simulink model "Weight_Extract_IQRD_RLS_model_top_8x8"  (R2020b)
settings: Solver=VariableStepAuto  StartTime=0.0  StopTime=0.00001  RelTol=1e-3
settings Model: Creator=jgentile  LastModifiedBy=jgentile

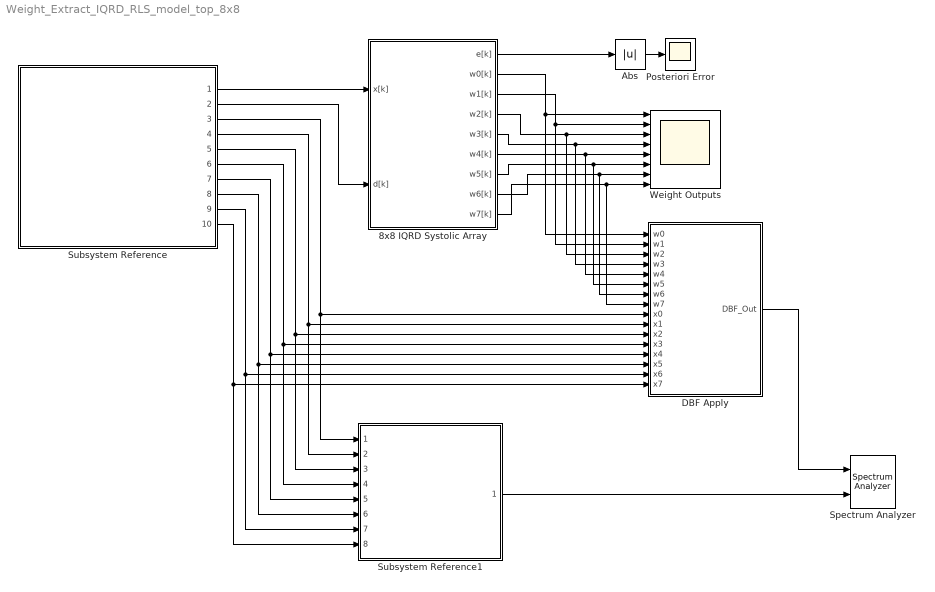
== system Weight_Extract_IQRD_RLS_model_top_8x8 ==
  8x8 IQRD Systolic Array : Subsystem
  Abs : Abs
  DBF Apply : Subsystem
  Posteriori Error : Scope
  Spectrum Analyzer : SpectrumAnalyzer  NumInputPorts=2
  Subsystem Reference : Subsystem  ReferencedSubsystem=s8x8_ULA_additive_Noise_Interference
  Subsystem Reference1 : Subsystem  ReferencedSubsystem=Weighted_Sum_Avg_No_ABF_8x8
  Weight Outputs : Scope  NumInputPorts=8
  wires:
  Subsystem Reference/1 -> 8x8 IQRD Systolic Array/1(x[k])
  Subsystem Reference/2 -> 8x8 IQRD Systolic Array/2(d[k])
  8x8 IQRD Systolic Array/2(w0[k]) -> DBF Apply/1(w0), Weight Outputs/1
  8x8 IQRD Systolic Array/3(w1[k]) -> DBF Apply/2(w1), Weight Outputs/2
  8x8 IQRD Systolic Array/4(w2[k]) -> DBF Apply/3(w2), Weight Outputs/3
  Subsystem Reference1/1 -> Spectrum Analyzer/2
  DBF Apply/1(DBF_Out) -> Spectrum Analyzer/1
  Abs/1 -> Posteriori Error/1
  Subsystem Reference/3 -> DBF Apply/9(x0), Subsystem Reference1/1
  Subsystem Reference/4 -> DBF Apply/10(x1), Subsystem Reference1/2
  Subsystem Reference/5 -> DBF Apply/11(x2), Subsystem Reference1/3
  Subsystem Reference/6 -> DBF Apply/12(x3), Subsystem Reference1/4
  Subsystem Reference/7 -> DBF Apply/13(x4), Subsystem Reference1/5
  Subsystem Reference/8 -> DBF Apply/14(x5), Subsystem Reference1/6
  Subsystem Reference/9 -> DBF Apply/15(x6), Subsystem Reference1/7
  Subsystem Reference/10 -> DBF Apply/16(x7), Subsystem Reference1/8
  8x8 IQRD Systolic Array/1(e[k]) -> Abs/1
  8x8 IQRD Systolic Array/5(w3[k]) -> DBF Apply/4(w3), Weight Outputs/4
  8x8 IQRD Systolic Array/6(w4[k]) -> DBF Apply/5(w4), Weight Outputs/5
  8x8 IQRD Systolic Array/7(w5[k]) -> DBF Apply/6(w5), Weight Outputs/6
  8x8 IQRD Systolic Array/8(w6[k]) -> DBF Apply/7(w6), Weight Outputs/7
  8x8 IQRD Systolic Array/9(w7[k]) -> DBF Apply/8(w7), Weight Outputs/8

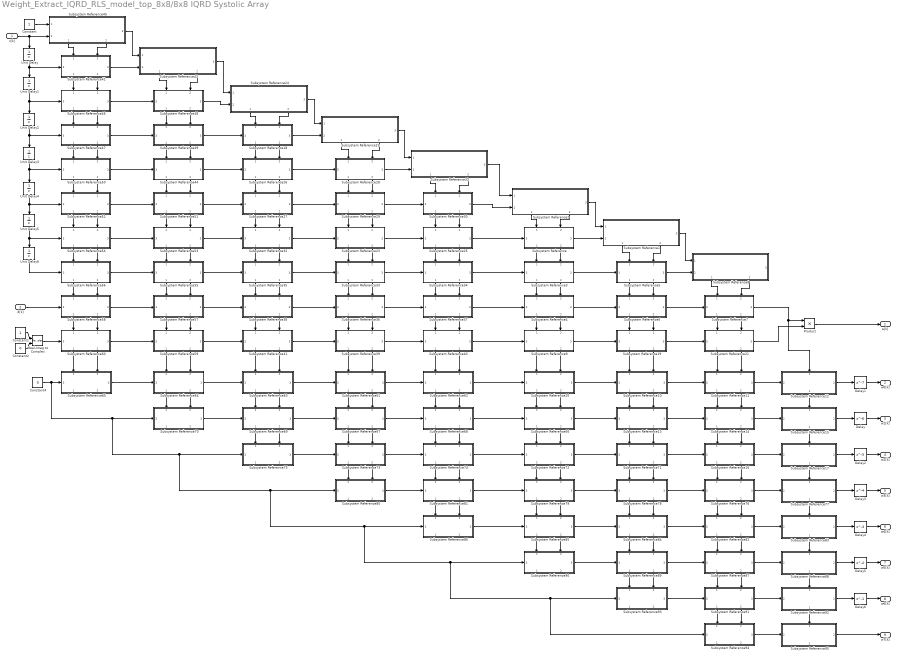
== system Weight_Extract_IQRD_RLS_model_top_8x8/8x8 IQRD Systolic Array ==
  x[k] : Inport
  d[k] : Inport  Port=2
  Constant : Constant
  Constant1 : Constant
  Constant2 : Constant  Value=0
  Constant4 : Constant  Value=0
  Delay : Delay  DelayLength=6
  Delay1 : Delay  DelayLength=7
  Delay2 : Delay  DelayLength=5
  Delay3 : Delay  DelayLength=4
  Delay4 : Delay  DelayLength=3
  Delay5 : Delay
  Delay6 : Delay  DelayLength=1
  Product : Product
  Real-Imag to Complex : RealImagToComplex
  Subsystem Reference{,3..7,9,18..19,21,23,25..30,32..42,44,46..60} (44 alike) : Subsystem  ReferencedSubsystem=internal_cell_givens
      settings: PortSchema="{\"entries\":[{\"content\":{\"sides\":[{\"content\":{\"connectorIds\":[\"In3\"]},\"type\":\"ConnectorPlacement.EquallySpacedRectSide\",\"uuid\":\"0239e4e7-44b6-4143-a587-38d4cded4ca6\"},{\"content\":{\"connectorIds\":[\"Out3\"],\"side\":\"RIGHT\"},\"type\":\"ConnectorPlacement.EquallySpacedRectSide\",\"uuid\":\"ea23c866-1a25-41e9-a0f2-3862af1c86e1\"},{\"content\":{\"connectorIds\":[\"In1\",\"In2\"],\"side\":\"TOP\"},\"type\":\"ConnectorPlacement.EquallySpacedRectSide\",\"uuid\":\"8a8bb13e-2e16-40e7-9ca3-19d820578314\"},{\"content\":{\"connectorIds\":[\"Out1\",\"Out2\"],\"side\":\"BOTTOM\"},\"type\":\"ConnectorPlacement.EquallySpacedRectSide\",\"uuid\":\"1be66ea9-adc8-4a43-a798-b14d6fcab7cd\"},{\"content\":{\"connectorIds\":[],\"side\":\"HIDDEN\"},\"type\":\"ConnectorPlacement.EquallySpacedRectSide\",\"uuid\":\"0fecdaf4-55de-420b-b554-931c979049af\"}]},\"type\":\"ConnectorPlacement.EquallySpacedConnector\",\"uuid\":\"70182f79-db57-400d-a53f-39946a20555a\"}],\"packageUris\":[\"http://schema.mathworks.com/mf0/Connector/R2020b\"],\"version\":\"1.0\"}"
  Subsystem Reference{1..2,8,22,24,31,43,45} (8 alike) : Subsystem  ReferencedSubsystem=boundary_cell_givens
      settings: PortSchema="{\"entries\":[{\"content\":{\"sides\":[{\"content\":{\"connectorIds\":[\"In1\",\"In2\"]},\"type\":\"ConnectorPlacement.EquallySpacedRectSide\",\"uuid\":\"11c023aa-376d-416d-bfcd-8d7843f2be22\"},{\"content\":{\"connectorIds\":[\"Out3\"],\"side\":\"RIGHT\"},\"type\":\"ConnectorPlacement.EquallySpacedRectSide\",\"uuid\":\"1a04016b-daba-4444-ad99-d7273a1feb5b\"},{\"content\":{\"connectorIds\":[],\"side\":\"TOP\"},\"type\":\"ConnectorPlacement.EquallySpacedRectSide\",\"uuid\":\"dd6dcf65-02b5-4ffa-b5ff-7e58c587941b\"},{\"content\":{\"connectorIds\":[\"Out1\",\"Out2\"],\"side\":\"BOTTOM\"},\"type\":\"ConnectorPlacement.EquallySpacedRectSide\",\"uuid\":\"26ecda3d-5bd8-4d7b-b858-e25b16c314b4\"},{\"content\":{\"connectorIds\":[],\"side\":\"HIDDEN\"},\"type\":\"ConnectorPlacement.EquallySpacedRectSide\",\"uuid\":\"bd7630cc-a9b8-4021-b6b5-0e32bd520d7d\"}]},\"type\":\"ConnectorPlacement.EquallySpacedConnector\",\"uuid\":\"7bb81265-b299-46b6-8c47-6bc2be69935c\"}],\"packageUris\":[\"http://schema.mathworks.com/mf0/Connector/R2020b\"],\"version\":\"1.0\"}"
  Subsystem Reference{10..11,13..14,16,20,61..76,78..82,84..87,89..91,93..94} (36 alike) : Subsystem  ReferencedSubsystem=inv_internal_cell_givens
      settings: PortSchema="{\"entries\":[{\"content\":{\"sides\":[{\"content\":{\"connectorIds\":[\"In3\"]},\"type\":\"ConnectorPlacement.EquallySpacedRectSide\",\"uuid\":\"7a30fd97-238e-4d3f-b86c-0b989816bca0\"},{\"content\":{\"connectorIds\":[\"Out3\"],\"side\":\"RIGHT\"},\"type\":\"ConnectorPlacement.EquallySpacedRectSide\",\"uuid\":\"97592077-7dd1-4e2a-9ce3-178c2c88f4d0\"},{\"content\":{\"connectorIds\":[\"In1\",\"In2\"],\"side\":\"TOP\"},\"type\":\"ConnectorPlacement.EquallySpacedRectSide\",\"uuid\":\"6aed6abb-33ac-4a40-86f4-2f1f080d5792\"},{\"content\":{\"connectorIds\":[\"Out1\",\"Out2\"],\"side\":\"BOTTOM\"},\"type\":\"ConnectorPlacement.EquallySpacedRectSide\",\"uuid\":\"d6ad6c95-90c4-469b-9aab-57bb42a059b1\"},{\"content\":{\"connectorIds\":[],\"side\":\"HIDDEN\"},\"type\":\"ConnectorPlacement.EquallySpacedRectSide\",\"uuid\":\"5567bba2-9935-40d2-a99a-4fbdd449a1bc\"}]},\"type\":\"ConnectorPlacement.EquallySpacedConnector\",\"uuid\":\"249ba23d-f701-4623-a398-9ae5c4f4b120\"}],\"packageUris\":[\"http://schema.mathworks.com/mf0/Connector/R2020b\"],\"version\":\"1.0\"}"
  Subsystem Reference{12,15,17,77,83,88,92,95} (8 alike) : Subsystem  ReferencedSubsystem=weight_extraction_cell
      settings: PortSchema="{\"entries\":[{\"content\":{\"sides\":[{\"content\":{\"connectorIds\":[\"In2\"]},\"type\":\"ConnectorPlacement.EquallySpacedRectSide\",\"uuid\":\"9b04af24-e055-4aa7-86bb-25e5a28bc350\"},{\"content\":{\"connectorIds\":[\"Out2\"],\"side\":\"RIGHT\"},\"type\":\"ConnectorPlacement.EquallySpacedRectSide\",\"uuid\":\"53a25428-f4c1-4318-807f-cb7f3198556b\"},{\"content\":{\"connectorIds\":[\"In1\"],\"side\":\"TOP\"},\"type\":\"ConnectorPlacement.EquallySpacedRectSide\",\"uuid\":\"c50d1458-d1ed-421b-b0d3-a6feb6118700\"},{\"content\":{\"connectorIds\":[\"Out1\"],\"side\":\"BOTTOM\"},\"type\":\"ConnectorPlacement.EquallySpacedRectSide\",\"uuid\":\"27032688-b9dc-465c-a4e2-c55a8672e920\"},{\"content\":{\"connectorIds\":[],\"side\":\"HIDDEN\"},\"type\":\"ConnectorPlacement.EquallySpacedRectSide\",\"uuid\":\"96ce2d10-4cc2-4967-91b3-9dd1803ae9a9\"}]},\"type\":\"ConnectorPlacement.EquallySpacedConnector\",\"uuid\":\"5dd7c3ab-20de-4667-a451-601882658f5a\"}],\"packageUris\":[\"http://schema.mathworks.com/mf0/Connector/R2020b\"],\"version\":\"1.0\"}"
  Unit Delay{,1..6} (7 alike) : UnitDelay  SampleTime=-1  HasFrameUpgradeWarning=on
  e[k] : Outport
  w0[k] : Outport  Port=2
  w1[k] : Outport  Port=3
  w2[k] : Outport  Port=4
  w3[k] : Outport  Port=5
  w4[k] : Outport  Port=6
  w5[k] : Outport  Port=7
  w6[k] : Outport  Port=8
  w7[k] : Outport  Port=9
  wires:
  Subsystem Reference2/1 -> Subsystem Reference/1
  Subsystem Reference1/1 -> Subsystem Reference5/1
  Subsystem Reference3/3 -> Subsystem Reference5/3
  Subsystem Reference/3 -> Subsystem Reference1/2
  Subsystem Reference4/3 -> Subsystem Reference6/3
  Subsystem Reference6/3 -> Subsystem Reference7/3
  x[k]/1 -> Subsystem Reference45/2, Unit Delay/1
  Subsystem Reference5/3 -> Subsystem Reference8/2
  Subsystem Reference3/2 -> Subsystem Reference4/2
  Subsystem Reference2/3 -> Subsystem Reference1/1
  Subsystem Reference/1 -> Subsystem Reference3/1
  Subsystem Reference3/1 -> Subsystem Reference4/1
  Subsystem Reference/2 -> Subsystem Reference3/2
  Subsystem Reference1/3 -> Subsystem Reference8/1
  Subsystem Reference5/2 -> Subsystem Reference6/2
  Subsystem Reference5/1 -> Subsystem Reference6/1
  Subsystem Reference2/2 -> Subsystem Reference/2
  Unit Delay/1 -> Subsystem Reference42/3, Unit Delay1/1
  Subsystem Reference8/2 -> Subsystem Reference7/2
  Subsystem Reference1/2 -> Subsystem Reference5/2
  Subsystem Reference8/1 -> Subsystem Reference7/1
  Subsystem Reference20/3 -> Subsystem Reference10/3
  Subsystem Reference10/3 -> Subsystem Reference11/3
  Subsystem Reference10/1 -> Subsystem Reference13/1
  Subsystem Reference10/2 -> Subsystem Reference13/2
  Subsystem Reference11/1 -> Subsystem Reference14/1
  Subsystem Reference11/2 -> Subsystem Reference14/2
  Subsystem Reference14/1 -> Subsystem Reference16/1
  Subsystem Reference14/2 -> Subsystem Reference16/2
  Subsystem Reference13/3 -> Subsystem Reference14/3
  Subsystem Reference15/2 -> Delay/1
  Delay/1 -> w1[k]/1
  Subsystem Reference12/2 -> Delay1/1
  Delay1/1 -> w0[k]/1
  Subsystem Reference19/3 -> Subsystem Reference21/3
  Subsystem Reference9/3 -> Subsystem Reference19/3
  Subsystem Reference4/1 -> Subsystem Reference9/1
  Subsystem Reference4/2 -> Subsystem Reference9/2
  Subsystem Reference6/1 -> Subsystem Reference19/1
  Subsystem Reference6/2 -> Subsystem Reference19/2
  Subsystem Reference7/1 -> Subsystem Reference21/1
  Subsystem Reference7/2 -> Subsystem Reference21/2
  Constant1/1 -> Real-Imag to Complex/1
  Constant2/1 -> Real-Imag to Complex/2
  Subsystem Reference9/1 -> Subsystem Reference20/1
  Subsystem Reference9/2 -> Subsystem Reference20/2
  Subsystem Reference19/1 -> Subsystem Reference10/1
  Subsystem Reference19/2 -> Subsystem Reference10/2
  Subsystem Reference21/1 -> Subsystem Reference11/1
  Subsystem Reference21/2 -> Subsystem Reference11/2
  Subsystem Reference11/3 -> Subsystem Reference12/2
  Subsystem Reference14/3 -> Subsystem Reference15/2
  Subsystem Reference16/3 -> Subsystem Reference17/2
  Subsystem Reference12/1 -> Subsystem Reference15/1
  Subsystem Reference15/1 -> Subsystem Reference17/1
  Subsystem Reference7/3 -> Subsystem Reference12/1, Product/1
  Subsystem Reference21/3 -> Product/2
  Product/1 -> e[k]/1
  Subsystem Reference30/1 -> Subsystem Reference25/1
  Subsystem Reference29/2 -> Subsystem Reference23/2
  Subsystem Reference29/1 -> Subsystem Reference23/1
  Subsystem Reference27/2 -> Subsystem Reference32/2
  Subsystem Reference27/1 -> Subsystem Reference32/1
  Subsystem Reference31/1 -> Subsystem Reference30/1
  Subsystem Reference22/2 -> Subsystem Reference28/2
  Subsystem Reference24/2 -> Subsystem Reference18/2
  Subsystem Reference28/1 -> Subsystem Reference29/1
  Subsystem Reference28/2 -> Subsystem Reference29/2
  Subsystem Reference22/3 -> Subsystem Reference31/1
  Subsystem Reference18/2 -> Subsystem Reference26/2
  Subsystem Reference26/1 -> Subsystem Reference27/1
  Subsystem Reference18/1 -> Subsystem Reference26/1
  Subsystem Reference24/3 -> Subsystem Reference22/1
  Subsystem Reference26/2 -> Subsystem Reference27/2
  Subsystem Reference28/3 -> Subsystem Reference31/2
  Subsystem Reference29/3 -> Subsystem Reference30/3
  Subsystem Reference27/3 -> Subsystem Reference29/3
  Subsystem Reference18/3 -> Subsystem Reference22/2
  Subsystem Reference26/3 -> Subsystem Reference28/3
  Subsystem Reference22/1 -> Subsystem Reference28/1
  Subsystem Reference24/1 -> Subsystem Reference18/1
  Subsystem Reference25/3 -> Subsystem Reference/3
  Subsystem Reference30/3 -> Subsystem Reference2/2
  Subsystem Reference30/2 -> Subsystem Reference25/2
  Subsystem Reference31/2 -> Subsystem Reference30/2
  Subsystem Reference31/3 -> Subsystem Reference2/1
  Subsystem Reference45/1 -> Subsystem Reference42/1
  Subsystem Reference43/1 -> Subsystem Reference48/1
  Subsystem Reference46/3 -> Subsystem Reference48/3
  Subsystem Reference42/3 -> Subsystem Reference43/2
  Subsystem Reference47/3 -> Subsystem Reference49/3
  Subsystem Reference46/2 -> Subsystem Reference47/2
  Subsystem Reference45/3 -> Subsystem Reference43/1
  Subsystem Reference42/1 -> Subsystem Reference46/1
  Subsystem Reference46/1 -> Subsystem Reference47/1
  Subsystem Reference42/2 -> Subsystem Reference46/2
  Subsystem Reference48/2 -> Subsystem Reference49/2
  Subsystem Reference48/1 -> Subsystem Reference49/1
  Subsystem Reference45/2 -> Subsystem Reference42/2
  Subsystem Reference43/2 -> Subsystem Reference48/2
  Subsystem Reference47/1 -> Subsystem Reference50/1
  Subsystem Reference47/2 -> Subsystem Reference50/2
  Subsystem Reference49/1 -> Subsystem Reference44/1
  Subsystem Reference49/2 -> Subsystem Reference44/2
  Subsystem Reference43/3 -> Subsystem Reference24/1
  Subsystem Reference48/3 -> Subsystem Reference24/2
  Subsystem Reference49/3 -> Subsystem Reference18/3
  Subsystem Reference44/3 -> Subsystem Reference26/3
  Subsystem Reference51/3 -> Subsystem Reference27/3
  Subsystem Reference53/3 -> Subsystem Reference32/3
  Subsystem Reference55/3 -> Subsystem Reference35/3
  Subsystem Reference50/3 -> Subsystem Reference44/3
  Subsystem Reference52/3 -> Subsystem Reference51/3
  Subsystem Reference54/3 -> Subsystem Reference53/3
  Subsystem Reference56/3 -> Subsystem Reference55/3
  Subsystem Reference58/3 -> Subsystem Reference57/3
  Subsystem Reference60/3 -> Subsystem Reference59/3
  Subsystem Reference50/1 -> Subsystem Reference52/1
  Subsystem Reference50/2 -> Subsystem Reference52/2
  Subsystem Reference52/1 -> Subsystem Reference54/1
  Subsystem Reference52/2 -> Subsystem Reference54/2
  Subsystem Reference54/1 -> Subsystem Reference56/1
  Subsystem Reference54/2 -> Subsystem Reference56/2
  Subsystem Reference56/1 -> Subsystem Reference58/1
  Subsystem Reference56/2 -> Subsystem Reference58/2
  Subsystem Reference58/1 -> Subsystem Reference60/1
  Subsystem Reference58/2 -> Subsystem Reference60/2
  Subsystem Reference44/1 -> Subsystem Reference51/1
  Subsystem Reference44/2 -> Subsystem Reference51/2
  Subsystem Reference51/1 -> Subsystem Reference53/1
  Subsystem Reference51/2 -> Subsystem Reference53/2
  Subsystem Reference53/1 -> Subsystem Reference55/1
  Subsystem Reference53/2 -> Subsystem Reference55/2
  Subsystem Reference55/1 -> Subsystem Reference57/1
  Subsystem Reference55/2 -> Subsystem Reference57/2
  Subsystem Reference57/1 -> Subsystem Reference59/1
  Subsystem Reference57/2 -> Subsystem Reference59/2
  Subsystem Reference57/3 -> Subsystem Reference38/3
  Subsystem Reference59/3 -> Subsystem Reference41/3
  Subsystem Reference32/3 -> Subsystem Reference23/3
  Subsystem Reference35/3 -> Subsystem Reference33/3
  Subsystem Reference38/3 -> Subsystem Reference36/3
  Subsystem Reference41/3 -> Subsystem Reference39/3
  Subsystem Reference32/1 -> Subsystem Reference35/1
  Subsystem Reference32/2 -> Subsystem Reference35/2
  Subsystem Reference35/1 -> Subsystem Reference38/1
  Subsystem Reference35/2 -> Subsystem Reference38/2
  Subsystem Reference38/1 -> Subsystem Reference41/1
  Subsystem Reference38/2 -> Subsystem Reference41/2
  Subsystem Reference23/3 -> Subsystem Reference25/3
  Subsystem Reference33/3 -> Subsystem Reference34/3
  Subsystem Reference23/1 -> Subsystem Reference33/1
  Subsystem Reference23/2 -> Subsystem Reference33/2
  Subsystem Reference33/1 -> Subsystem Reference36/1
  Subsystem Reference33/2 -> Subsystem Reference36/2
  Subsystem Reference36/1 -> Subsystem Reference39/1
  Subsystem Reference36/2 -> Subsystem Reference39/2
  Subsystem Reference36/3 -> Subsystem Reference37/3
  Subsystem Reference39/3 -> Subsystem Reference40/3
  Subsystem Reference25/1 -> Subsystem Reference34/1
  Subsystem Reference25/2 -> Subsystem Reference34/2
  Subsystem Reference34/1 -> Subsystem Reference37/1
  Subsystem Reference34/2 -> Subsystem Reference37/2
  Subsystem Reference37/1 -> Subsystem Reference40/1
  Subsystem Reference37/2 -> Subsystem Reference40/2
  Subsystem Reference34/3 -> Subsystem Reference3/3
  Subsystem Reference37/3 -> Subsystem Reference4/3
  Subsystem Reference40/3 -> Subsystem Reference9/3
  Subsystem Reference40/2 -> Subsystem Reference62/2
  Subsystem Reference40/1 -> Subsystem Reference62/1
  Subsystem Reference39/2 -> Subsystem Reference61/2
  Subsystem Reference39/1 -> Subsystem Reference61/1
  Subsystem Reference41/2 -> Subsystem Reference63/2
  Subsystem Reference41/1 -> Subsystem Reference63/1
  Subsystem Reference61/3 -> Subsystem Reference62/3
  Subsystem Reference63/3 -> Subsystem Reference61/3
  Subsystem Reference62/3 -> Subsystem Reference20/3
  Subsystem Reference65/3 -> Subsystem Reference64/3
  Subsystem Reference60/1 -> Subsystem Reference65/1
  Subsystem Reference60/2 -> Subsystem Reference65/2
  Subsystem Reference59/1 -> Subsystem Reference64/1
  Subsystem Reference59/2 -> Subsystem Reference64/2
  Subsystem Reference64/3 -> Subsystem Reference63/3
  Subsystem Reference70/3 -> Subsystem Reference69/3
  Subsystem Reference68/3 -> Subsystem Reference66/3
  Subsystem Reference69/3 -> Subsystem Reference67/3
  Subsystem Reference67/3 -> Subsystem Reference68/3
  Subsystem Reference66/3 -> Subsystem Reference13/3
  Subsystem Reference72/3 -> Subsystem Reference71/3
  Subsystem Reference73/3 -> Subsystem Reference74/3
  Subsystem Reference75/3 -> Subsystem Reference73/3
  Subsystem Reference74/3 -> Subsystem Reference72/3
  Subsystem Reference71/3 -> Subsystem Reference16/3
  Subsystem Reference17/2 -> Delay2/1
  Delay2/1 -> w2[k]/1
  Delay3/1 -> w3[k]/1
  Subsystem Reference77/2 -> Delay3/1
  Subsystem Reference78/3 -> Subsystem Reference76/3
  Subsystem Reference81/3 -> Subsystem Reference79/3
  Subsystem Reference80/3 -> Subsystem Reference81/3
  Subsystem Reference79/3 -> Subsystem Reference78/3
  Subsystem Reference76/3 -> Subsystem Reference77/2
  Subsystem Reference82/3 -> Subsystem Reference83/2
  Subsystem Reference85/3 -> Subsystem Reference84/3
  Subsystem Reference86/3 -> Subsystem Reference85/3
  Subsystem Reference84/3 -> Subsystem Reference82/3
  Subsystem Reference83/2 -> Delay4/1
  Delay4/1 -> w4[k]/1
  Delay5/1 -> w5[k]/1
  Subsystem Reference88/2 -> Delay5/1
  Subsystem Reference89/3 -> Subsystem Reference87/3
  Subsystem Reference90/3 -> Subsystem Reference89/3
  Subsystem Reference87/3 -> Subsystem Reference88/2
  Subsystem Reference91/3 -> Subsystem Reference92/2
  Subsystem Reference93/3 -> Subsystem Reference91/3
  Subsystem Reference92/2 -> Delay6/1
  Delay6/1 -> w6[k]/1
  Subsystem Reference95/2 -> w7[k]/1
  Subsystem Reference94/3 -> Subsystem Reference95/2
  Constant4/1 -> Subsystem Reference94/3, Subsystem Reference93/3, Subsystem Reference90/3, Subsystem Reference86/3, Subsystem Reference80/3, Subsystem Reference75/3, Subsystem Reference70/3, Subsystem Reference65/3
  Subsystem Reference64/1 -> Subsystem Reference70/1
  Subsystem Reference64/2 -> Subsystem Reference70/2
  Subsystem Reference63/1 -> Subsystem Reference69/1
  Subsystem Reference63/2 -> Subsystem Reference69/2
  Subsystem Reference69/1 -> Subsystem Reference75/1
  Subsystem Reference69/2 -> Subsystem Reference75/2
  Subsystem Reference61/1 -> Subsystem Reference67/1
  Subsystem Reference61/2 -> Subsystem Reference67/2
  Subsystem Reference67/1 -> Subsystem Reference73/1
  Subsystem Reference67/2 -> Subsystem Reference73/2
  Subsystem Reference73/1 -> Subsystem Reference80/1
  Subsystem Reference73/2 -> Subsystem Reference80/2
  Subsystem Reference62/1 -> Subsystem Reference68/1
  Subsystem Reference62/2 -> Subsystem Reference68/2
  Subsystem Reference68/1 -> Subsystem Reference74/1
  Subsystem Reference68/2 -> Subsystem Reference74/2
  Subsystem Reference74/1 -> Subsystem Reference81/1
  Subsystem Reference74/2 -> Subsystem Reference81/2
  Subsystem Reference81/1 -> Subsystem Reference86/1
  Subsystem Reference81/2 -> Subsystem Reference86/2
  Subsystem Reference20/1 -> Subsystem Reference66/1
  Subsystem Reference20/2 -> Subsystem Reference66/2
  Subsystem Reference66/1 -> Subsystem Reference72/1
  Subsystem Reference66/2 -> Subsystem Reference72/2
  Subsystem Reference72/1 -> Subsystem Reference79/1
  Subsystem Reference72/2 -> Subsystem Reference79/2
  Subsystem Reference79/1 -> Subsystem Reference85/1
  Subsystem Reference79/2 -> Subsystem Reference85/2
  Subsystem Reference85/1 -> Subsystem Reference90/1
  Subsystem Reference85/2 -> Subsystem Reference90/2
  Subsystem Reference13/1 -> Subsystem Reference71/1
  Subsystem Reference13/2 -> Subsystem Reference71/2
  Subsystem Reference71/1 -> Subsystem Reference78/1
  Subsystem Reference71/2 -> Subsystem Reference78/2
  Subsystem Reference78/1 -> Subsystem Reference84/1
  Subsystem Reference78/2 -> Subsystem Reference84/2
  Subsystem Reference84/1 -> Subsystem Reference89/1
  Subsystem Reference84/2 -> Subsystem Reference89/2
  Subsystem Reference89/1 -> Subsystem Reference93/1
  Subsystem Reference89/2 -> Subsystem Reference93/2
  Subsystem Reference16/1 -> Subsystem Reference76/1
  Subsystem Reference16/2 -> Subsystem Reference76/2
  Subsystem Reference17/1 -> Subsystem Reference77/1
  Subsystem Reference76/1 -> Subsystem Reference82/1
  Subsystem Reference76/2 -> Subsystem Reference82/2
  Subsystem Reference77/1 -> Subsystem Reference83/1
  Subsystem Reference82/1 -> Subsystem Reference87/1
  Subsystem Reference82/2 -> Subsystem Reference87/2
  Subsystem Reference83/1 -> Subsystem Reference88/1
  Subsystem Reference87/1 -> Subsystem Reference91/1
  Subsystem Reference87/2 -> Subsystem Reference91/2
  Subsystem Reference88/1 -> Subsystem Reference92/1
  Subsystem Reference91/1 -> Subsystem Reference94/1
  Subsystem Reference91/2 -> Subsystem Reference94/2
  Subsystem Reference92/1 -> Subsystem Reference95/1
  Real-Imag to Complex/1 -> Subsystem Reference60/3
  d[k]/1 -> Subsystem Reference58/3
  Constant/1 -> Subsystem Reference45/1
  Unit Delay6/1 -> Subsystem Reference56/3
  Unit Delay5/1 -> Unit Delay6/1, Subsystem Reference54/3
  Unit Delay4/1 -> Unit Delay5/1, Subsystem Reference52/3
  Unit Delay3/1 -> Unit Delay4/1, Subsystem Reference50/3
  Unit Delay2/1 -> Unit Delay3/1, Subsystem Reference47/3
  Unit Delay1/1 -> Unit Delay2/1, Subsystem Reference46/3

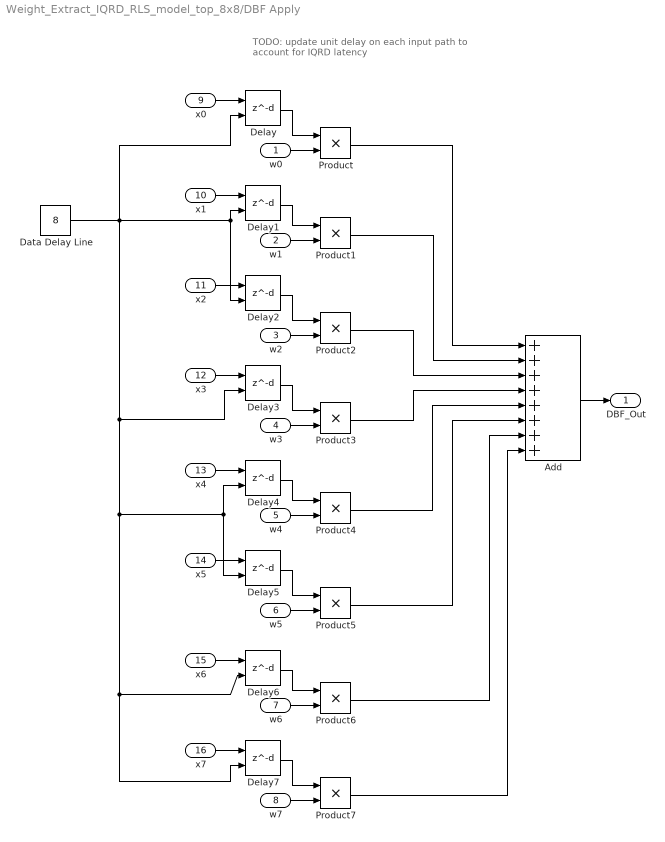
== system Weight_Extract_IQRD_RLS_model_top_8x8/DBF Apply ==
  note: TODO: update unit delay on each input path
      | to account for IQRD latency
  w0 : Inport
  w1 : Inport  Port=2
  w2 : Inport  Port=3
  w3 : Inport  Port=4
  w4 : Inport  Port=5
  w5 : Inport  Port=6
  w6 : Inport  Port=7
  w7 : Inport  Port=8
  x0 : Inport  Port=9
  x1 : Inport  Port=10
  x2 : Inport  Port=11
  x3 : Inport  Port=12
  x4 : Inport  Port=13
  x5 : Inport  Port=14
  x6 : Inport  Port=15
  x7 : Inport  Port=16
  Add : Sum  Inputs=++++++++
  Data Delay Line : Constant  Value=8
  Delay{,1..7} (8 alike) : Delay  DelayLengthSource=Input port
      settings: InputPortMap=u0,p1
  Product{,1..7} (8 alike) : Product
  DBF_Out : Outport
  wires:
  Delay1/1 -> Product1/1
  Add/1 -> DBF_Out/1
  w0/1 -> Product/2
  Delay/1 -> Product/1
  Product/1 -> Add/1
  x1/1 -> Delay1/1
  x2/1 -> Delay2/1
  w1/1 -> Product1/2
  w2/1 -> Product2/2
  x0/1 -> Delay/1
  Delay2/1 -> Product2/1
  Product2/1 -> Add/3
  Product1/1 -> Add/2
  Delay5/1 -> Product5/1
  x3/1 -> Delay3/1
  w5/1 -> Product5/2
  w4/1 -> Product4/2
  x5/1 -> Delay5/1
  x4/1 -> Delay4/1
  Delay3/1 -> Product3/1
  w3/1 -> Product3/2
  Delay4/1 -> Product4/1
  Data Delay Line/1 -> Delay3/2, Delay4/2, Delay5/2, Delay6/2, Delay7/2, Delay2/2, Delay1/2, Delay/2
  Delay6/1 -> Product6/1
  x6/1 -> Delay6/1
  x7/1 -> Delay7/1
  w6/1 -> Product6/2
  w7/1 -> Product7/2
  Delay7/1 -> Product7/1
  Product3/1 -> Add/4
  Product4/1 -> Add/5
  Product5/1 -> Add/6
  Product6/1 -> Add/7
  Product7/1 -> Add/8
